simulink model "KS_HF_fixed"  (R2023b)
settings: Solver=FixedStepAuto  StartTime=0.0  StopTime=15  RelTol=1e-3
values from neighbouring files (symbols this model uses):
  period_sequence = normalised_period(f_s,input_seq)    [main.m]
  playback_speed = 0.5    [main.m]
  T_s = 1/f_s    (= 9.07029478458e-05)    [main.m]
undefined symbols (not defined in the file or in its folder): gaussian
libraries: simulink x3, dspsrcs4 x1, dspvision x1
settings Model: CodeVerificationMode=processor-in-the-loop (pil)  Creator=andre  LastModifiedBy=Rorya
settings OptimizationCC: DefaultParameterBehavior=Inlined  EnhancedBackFolding=on  PassReuseOutputArgsAs=Individual arguments  ZeroExternalMemoryAtStartup=off  ZeroInternalMemoryAtStartup=off  OptimizeBlockOrder=speed  DifferentSizesBufferReuse=on  OptimizationCustomize=off  EfficientTunableParamExpr=on
settings DebuggingCC: ParameterTunabilityLossMsg=error
settings SFSimCC: MATLABDynamicMemAlloc=off
settings RTWCC: Description=Embedded Coder  SystemTargetFile=ert.tlc  TemplateMakefile=ert_default_tmf  GenerateReport=on  LaunchReport=on  CodeExecutionProfiling=on  CodeProfilingSaveOptions=AllData  CodeProfilingInstrumentation=detailed  GenerateWebview=on  GenerateCodeMetricsReport=on
settings CodeAppCC: ForceParamTrailComments=on  IgnoreCustomStorageClasses=off  OperatorAnnotations=on  SimulinkDataObjDesc=on  SFDataObjDesc=on  InsertBlockDesc=on
settings ERTTargetCC: TargetLangStandard=C99 (ISO)  GenerateSampleERTMain=on  InlinedParameterPlacement=NonHierarchical  ERTCustomFileTemplate=example_file_process.tlc

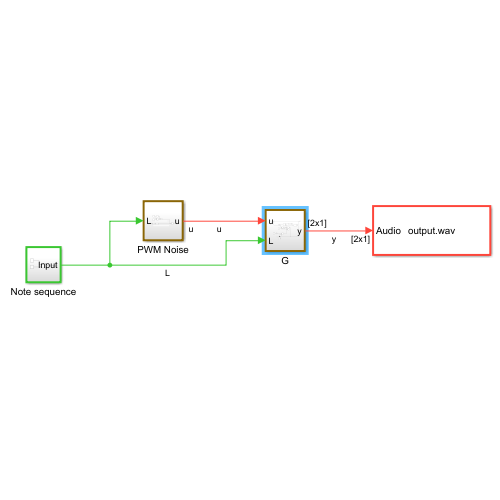
[thumbnail: Simulink's stored preview of the top-level diagram]
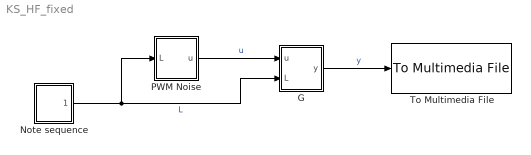
== system KS_HF_fixed ==
  G : Subsystem
  Note sequence : Subsystem
  PWM Noise : Subsystem
  To Multimedia File : dspvision/To Multimedia File  outputFilename=output.wav  streamSelection=Audio only  videoCompressor=None (uncompressed)  audioCompressor=None (uncompressed)  imagePorts=Separate color signals  fileType=WAV  audioDatatype=16-bit integer  fourcc=RGB  videoQuality=75  mj2000CompFactor=10
      settings: LibrarySourceBlock=dspsnks4/To Multimedia File
  wires:
  PWM Noise/1(u) -> G/1(u)  "u"
  Note sequence/1(Input) -> PWM Noise/1(L), G/2(L)  "L"
  G/1(y) -> To Multimedia File/1  "y"

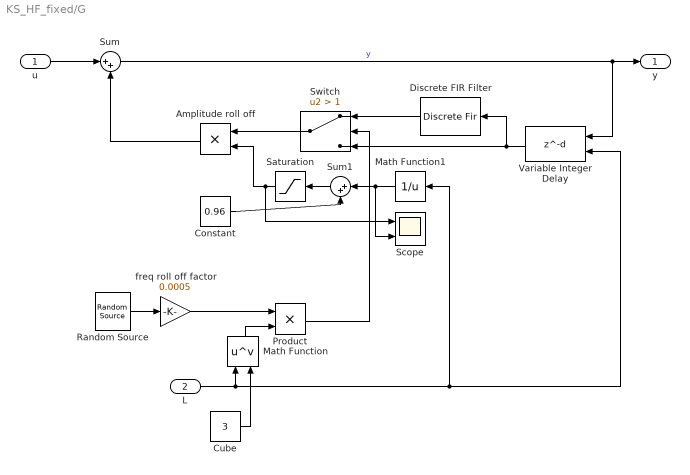
== system KS_HF_fixed/G ==
  u : Inport
  L : Inport  Port=2
  Amplitude roll off : Product
  Constant : Constant  Value=0.96
  Cube : Constant  Value=3
  Discrete FIR Filter : DiscreteFir
  Math Function : Math  Operator=pow
  Math Function1 : Math  Operator=reciprocal
  Product : Product
  Random Source : dspsrcs4/Random Source  SrcType=Uniform  NormMethod=Ziggurat  CltLength=12  MinVal=0  MaxVal=1  MeanVal=S_factor  VarVal=1  RepMode=Not repeatable  rawSeed=1  IsInherit=off  SampMode=Discrete  SampTime=T_s  SampFrame=1  DataType=Double  OutComplex=Real  OutputFrames=off
  Saturation : Saturate  UpperLimit=1  LowerLimit=0
  Scope : Scope  NumInputPorts=2
  Sum : Sum  Inputs=|++
  Sum1 : Sum  Inputs=|++
  Switch : Switch  Criteria=u2 > Threshold  Threshold=1  SaturateOnIntegerOverflow=off  InputSameDT=off
  Variable Integer Delay : Delay  DelayLengthSource=Input port  DelayLengthUpperLimit=256  PreventDirectFeedthrough=on  UseCircularBuffer=on
      settings: InputPortMap=u0,p1
  freq roll off factor : Gain  Gain=0.0005
  y : Outport
  wires:
  Amplitude roll off/1 -> Sum/2
  Sum/1 -> y/1, Variable Integer Delay/1  "y"
  u/1 -> Sum/1
  Switch/1 -> Amplitude roll off/1
  Product/1 -> Switch/2
  Discrete FIR Filter/1 -> Switch/1
  Variable Integer Delay/1 -> Switch/3, Discrete FIR Filter/1
  Math Function/1 -> Product/2
  freq roll off factor/1 -> Product/1
  Random Source/1 -> freq roll off factor/1
  Cube/1 -> Math Function/2
  Sum1/1 -> Saturation/1
  Constant/1 -> Sum1/2
  L/1 -> Math Function1/1, Variable Integer Delay/2, Math Function/1
  Math Function1/1 -> Sum1/1, Scope/2
  Saturation/1 -> Scope/1, Amplitude roll off/2

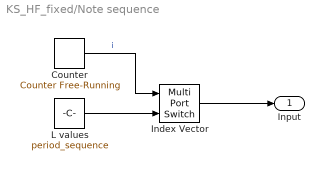
== system KS_HF_fixed/Note sequence ==
  Counter : simulink/Sources/Counter Free-Running  NumBits=seq_length  tsamp=playback_speed
  Index Vector : MultiPortSwitch  DataPortOrder=Zero-based contiguous  Inputs=1  zeroidx=on  SaturateOnIntegerOverflow=off  InputSameDT=off
  L values : Constant  Value=period_sequence
  Input : Outport
  wires:
  L values/1 -> Index Vector/2
  Index Vector/1 -> Input/1
  Counter/1 -> Index Vector/1  "i"

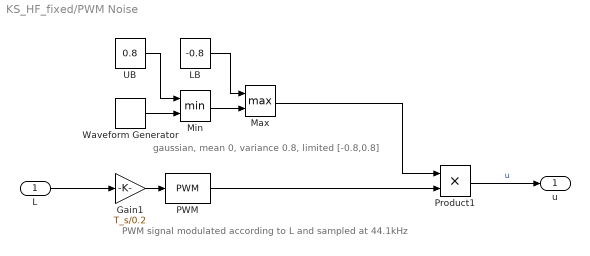
== system KS_HF_fixed/PWM Noise ==
  note: PWM signal modulated according to L and sampled at 44.1kHz
  note: gaussian, mean 0, variance 0.8, limited [-0.8,0.8]
  L : Inport
  Gain1 : Gain  Gain=T_s/0.2
  LB : Constant  Value=-0.8
  Max : MinMax  Function=max  Inputs=2
  Min : MinMax  Inputs=2
  PWM : simulink/Discontinuities/PWM  DisableCoverage=on  Period=playback_speed  InitialDelay=0  DisallowZeroDutyCycle=off  RunAtFixedTimeIntervals=on  SampleTime=T_s
  Product1 : Product
  UB : Constant  Value=0.8
  Waveform Generator : simulink/Sources/Waveform Generator  OutMin=[]  OutMax=[]  OutDataTypeStr=double  SelectedSignal=1  Signals=gaussian('Mean',0,'Variance',0.8,'Seed',1)  BlockNames=MultiportSwitch_c96a69a61ea7450  SampleTime=T_s
  u : Outport
  wires:
  LB/1 -> Max/1
  Waveform Generator/1 -> Min/2
  UB/1 -> Min/1
  Min/1 -> Max/2
  PWM/1 -> Product1/2
  Gain1/1 -> PWM/1
  L/1 -> Gain1/1
  Product1/1 -> u/1  "u"
  Max/1 -> Product1/1
